simulink model "Motion_trajectory"  (R2021b)
settings: Solver=ode4  StartTime=0.0  StopTime=25  FixedStep=1e-4  RelTol=1e-3
settings Model: Creator=francescoiotti  LastModifiedBy=vince

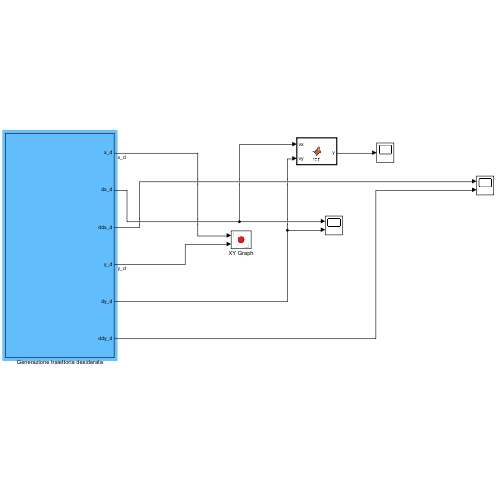
[thumbnail: Simulink's stored preview of the top-level diagram]
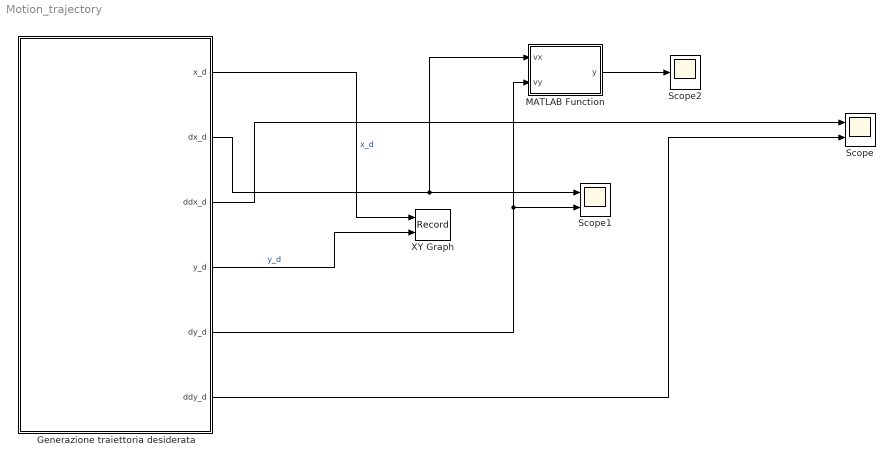
== system Motion_trajectory ==
  Generazione traiettoria desiderata : Subsystem
  MATLAB Function : MATLAB Function  TreatAsAtomicUnit=on
  Scope : Scope  NumInputPorts=2
  Scope1 : Scope  NumInputPorts=2
  Scope2 : Scope
  XY Graph : Record  FileSettingsInternal="{\"entries\":[{\"content\":{\"excelSettings\":{\"content\":{},\"type\":\"Streamout.ExcelSettings\"}},\"type\":\"Streamout.FileSettingStorage\",\"uuid\":\"cacf0d3f-48de-49d9-b0d8-d3cb2fe7912c\"}],\"packageUris\":[\"http://schema.mathworks.com/mf0/streamout_blocks/R2020a\"],\"version\":\"1.0\"}"  Layout=[1 1]  SignalsInternal="{\"entries\":[{\"content\":{\"signals\":[{\"content\":{\"blockPath\":[\"Motion_trajectory/XY Graph\"],\"channel\":[],\"dimensions\":[1],\"domain\":\"Motion_trajectory/XY Graph\",\"lineColor\":\"#a2142f\",\"plots\":[1],\"port\":1,\"sid\":[\"\"],\"signalID\":13129,\"signalName\":\"x_d\"},\"type\":\"RecordBlkView.Signal\",\"uuid\":\"ed82738d-0513-4c64-a845-4b3271580369\"},{\"content\":{\"blockPath\":[\"Motion_trajectory/XY Graph\"],\"channel\":[],\"dimensions\":[1],\"domain\":\"Motion_trajectory/XY Graph\",\"lineColor\":\"#139fff\",\"plots\":[1],\"port\":2,\"sid\":[\"\"],\"signalID\":13133,\"signalName\":\"y_d\"},\"type\":\"RecordBlkView.Signal\",\"uuid\":\"74c5c851-1e34-4755-b9d4-55e17618f5be\"}]},\"type\":\"RecordBlkView.InputSignals\",\"uuid\":\"75954b28-79ce-4988-8223-6aebadd83403\"}],\"packageUris\":[\"http://schema.mathworks.com/mf0/streamout_blocks/R2020a\"],\"version\":\"1.0\"}"  VisualizationBindings="{\"xyplotplugin\":{\"info\":[{\"series\":[{\"bindingParametersList\":[{\"parameter\":\"X-Axis\",\"signalID\":13129,\"signalName\":\"x_d\"},{\"parameter\":\"Y-Axis\",\"signalID\":13133,\"signalName\":\"y_d\"}],\"seriesID\":24234}],\"subplotID\":1}]}}"  CompatibilityTag=XY
  wires:
  Generazione traiettoria desiderata/1(x_d) -> XY Graph/1  "x_d"
  Generazione traiettoria desiderata/4(y_d) -> XY Graph/2  "y_d"
  Generazione traiettoria desiderata/3(ddx_d) -> Scope/1
  Generazione traiettoria desiderata/6(ddy_d) -> Scope/2
  Generazione traiettoria desiderata/2(dx_d) -> Scope1/1, MATLAB Function/1(vx)
  Generazione traiettoria desiderata/5(dy_d) -> MATLAB Function/2(vy), Scope1/2
  MATLAB Function/1(y) -> Scope2/1

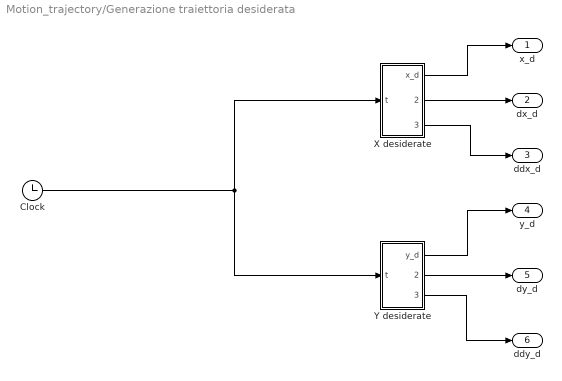
== system Motion_trajectory/Generazione traiettoria desiderata ==
  Clock : Clock
  X desiderate : Subsystem
  Y desiderate : Subsystem
  x_d : Outport
  dx_d : Outport  Port=2
  ddx_d : Outport  Port=3
  y_d : Outport  Port=4
  dy_d : Outport  Port=5
  ddy_d : Outport  Port=6
  wires:
  Y desiderate/1(y_d) -> y_d/1
  Y desiderate/2(dy_d) -> dy_d/1
  X desiderate/3(ddx_d) -> ddx_d/1
  X desiderate/2(dx_d) -> dx_d/1
  Y desiderate/3(ddy_d) -> ddy_d/1
  X desiderate/1(x_d) -> x_d/1
  Clock/1 -> X desiderate/1(t), Y desiderate/1(t)

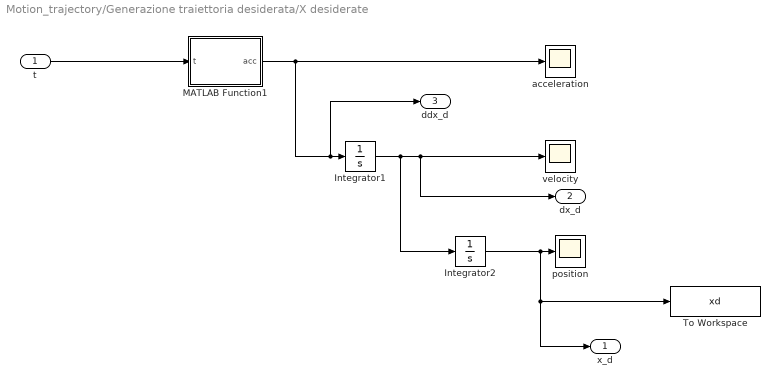
== system Motion_trajectory/Generazione traiettoria desiderata/X desiderate ==
  t : Inport
  Integrator1 : Integrator
  Integrator2 : Integrator
  MATLAB Function1 : MATLAB Function  TreatAsAtomicUnit=on
  To Workspace : ToWorkspace  VariableName=xd  SaveFormat=Structure  SampleTime=-1
  acceleration : Scope
  position : Scope
  velocity : Scope
  x_d : Outport
  dx_d : Outport  Port=2
  ddx_d : Outport  Port=3
  wires:
  MATLAB Function1/1(acc) -> acceleration/1, ddx_d/1, Integrator1/1
  t/1 -> MATLAB Function1/1(t)
  Integrator1/1 -> dx_d/1, velocity/1, Integrator2/1
  Integrator2/1 -> To Workspace/1, x_d/1, position/1

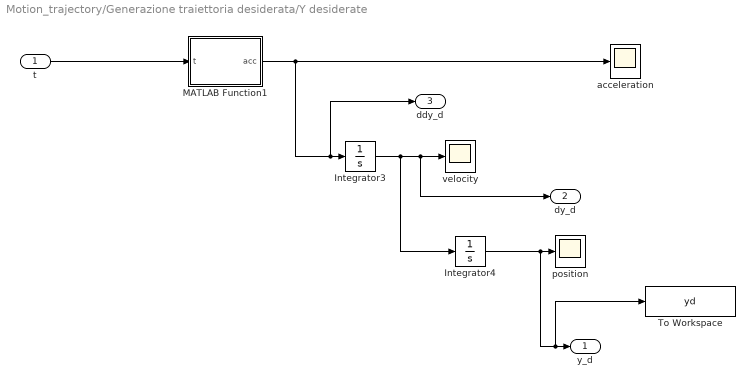
== system Motion_trajectory/Generazione traiettoria desiderata/Y desiderate ==
  t : Inport
  Integrator3 : Integrator
  Integrator4 : Integrator
  MATLAB Function1 : MATLAB Function  TreatAsAtomicUnit=on
  To Workspace : ToWorkspace  VariableName=yd  SaveFormat=Structure  SampleTime=-1
  acceleration : Scope
  position : Scope
  velocity : Scope
  y_d : Outport
  dy_d : Outport  Port=2
  ddy_d : Outport  Port=3
  wires:
  t/1 -> MATLAB Function1/1(t)
  MATLAB Function1/1(acc) -> Integrator3/1, ddy_d/1, acceleration/1
  Integrator3/1 -> velocity/1, dy_d/1, Integrator4/1
  Integrator4/1 -> position/1, To Workspace/1, y_d/1

== matlab function Motion_trajectory/MATLAB Function ==
  data: vx input; y output; vy input
function y = fcn(vx, vy)
v = [vx, vy];
y = norm(v);

== matlab function Motion_trajectory/Generazione traiettoria desiderata/Y desiderate/MATLAB Function1 ==
  data: t input; acc output
function acc = acceleration(t)
% Parametri
% a = 10*pi^4;
Ka = 1.75;
Kd = -1.75;
c1 = 2.5;
c2 = 5;
c3 = 7.5;
c4 = 10;

% Accelerating part
if t < c2
    a = Ka * exp(-(t-c1)^2/2);
% Decelerating part
% elseif t >= c1 && t < c2
%     a = Ka * exp(-(t-c2)^2/2);
% Decelerating part
elseif t >= c2 && t < c4 
    a = Kd * exp(-(t-c3)^2/2);
% Accelerating part
% elseif t >= c3 && t < c4
%     a = Kd * exp(-(t-c4)^2/2);
else
    a = 0;
end

acc = a;

== matlab function Motion_trajectory/Generazione traiettoria desiderata/X desiderate/MATLAB Function1 ==
  data: t input; acc output
function acc = acceleration(t)
% Parametri
% a = 10*pi^4;
Ka = 2.5;
Kd = -2.5;
c1 = 4;
c2 = 8;
c3 = 12;
c4 = 16;
c5 = 20;
c6 = 24;

% Accelerating part
if t < c2
    a = Ka * exp(-(t-c1)^2/2);

% Decelerating part
elseif t >= c2 && t < c3 
    a = Kd * exp(-(t-c3)^2/2);

% Inizio secondo picco di velocità
elseif t >= c3 && t < c4 
    a = 1.5 * exp(-(t-c3)^2/2);
% Decelero fino a fermarmi
elseif t >= c4 && t < c6 
    a = -1.5 * exp(-(t-c5)^2/2);
else
    a = 0;
end

acc = a;
